simulink model "drawing_only"  (R2022b)
settings: Solver=VariableStepAuto  StartTime=0.0  StopTime=160  RelTol=1e-3
libraries: fl_lib x8, simulink x1
settings Model: Creator=Haposan  LastModifiedBy=Haposan

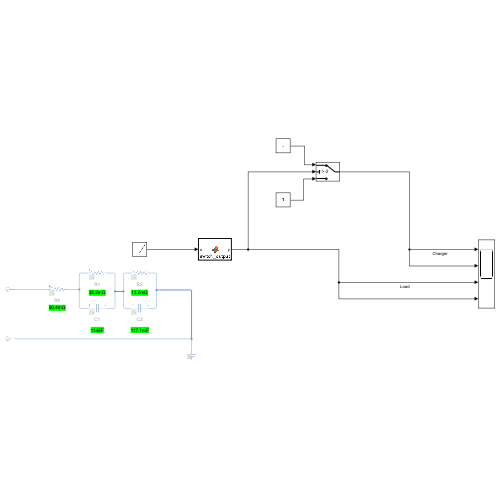
[thumbnail: Simulink's stored preview of the top-level diagram]
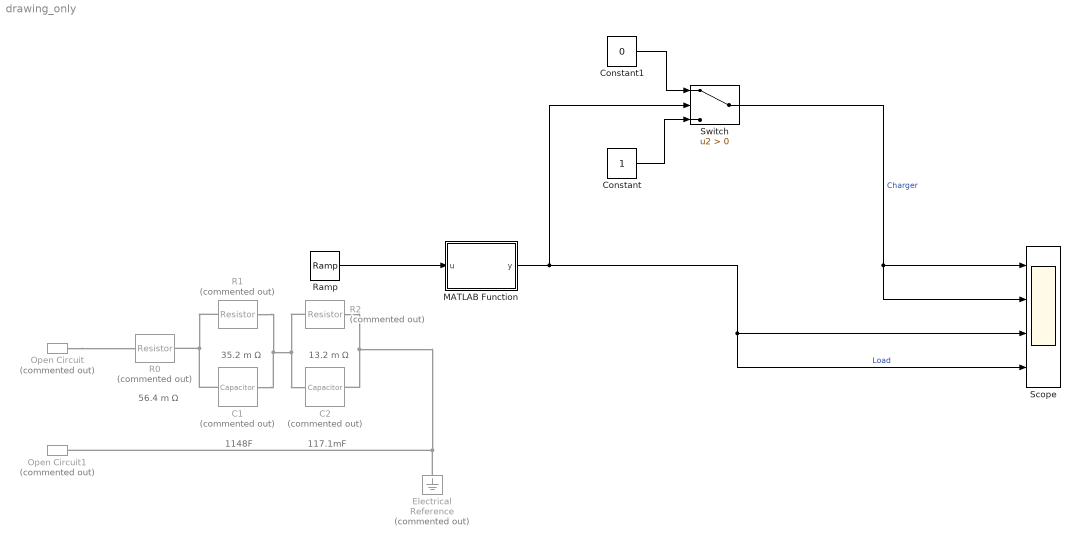
== system drawing_only ==
  note: 56.4 m Ω
  note: 13.2 m Ω
  note: 1148F
  note: 35.2 m Ω
  note: 117.1mF
  C1 : fl_lib/Electrical/Electrical Elements/Capacitor  Commented=on  c=1148 F  r=1e-6 Ohm  g=0 1/Ohm  i_specify=off  i_priority=None  i=0 A  i_nominal_specify=off  i_nominal_unit=A  i_nominal_value=1  v_specify=off  v_priority=None  v=0 V  v_nominal_specify=off  v_nominal_unit=V  v_nominal_value=1  vc_specify=off  vc_priority=High  vc=0 V  vc_nominal_specify=off  vc_nominal_unit=V  vc_nominal_value=1
  C2 : fl_lib/Electrical/Electrical Elements/Capacitor  Commented=on  c=117.1E-3 F  r=1e-6 Ohm  g=0 1/Ohm  i_specify=off  i_priority=None  i=0 A  i_nominal_specify=off  i_nominal_unit=A  i_nominal_value=1  v_specify=off  v_priority=None  v=0 V  v_nominal_specify=off  v_nominal_unit=V  v_nominal_value=1  vc_specify=off  vc_priority=High  vc=0 V  vc_nominal_specify=off  vc_nominal_unit=V  vc_nominal_value=1
  Constant : Constant
  Constant1 : Constant  Value=0
  Electrical Reference : fl_lib/Electrical/Electrical Elements/Electrical Reference  Commented=on
  MATLAB Function : MATLAB Function  TreatAsAtomicUnit=on
  Open Circuit : fl_lib/Electrical/Electrical Elements/Open Circuit  Commented=on  v_specify=off  v_priority=None  v=0 V  v_nominal_specify=off  v_nominal_unit=V  v_nominal_value=1
  Open Circuit1 : fl_lib/Electrical/Electrical Elements/Open Circuit  Commented=on  v_specify=off  v_priority=None  v=0 V  v_nominal_specify=off  v_nominal_unit=V  v_nominal_value=1
  R0 : fl_lib/Electrical/Electrical Elements/Resistor  Commented=on  R=56.4E-3 Ohm  i_specify=off  i_priority=None  i=0 A  i_nominal_specify=off  i_nominal_unit=A  i_nominal_value=1  v_specify=off  v_priority=None  v=0 V  v_nominal_specify=off  v_nominal_unit=V  v_nominal_value=1
  R1 : fl_lib/Electrical/Electrical Elements/Resistor  Commented=on  R=35.2E-3 Ohm  i_specify=off  i_priority=None  i=0 A  i_nominal_specify=off  i_nominal_unit=A  i_nominal_value=1  v_specify=off  v_priority=None  v=0 V  v_nominal_specify=off  v_nominal_unit=V  v_nominal_value=1
  R2 : fl_lib/Electrical/Electrical Elements/Resistor  Commented=on  R=13.2E-3 Ohm  i_specify=off  i_priority=None  i=0 A  i_nominal_specify=off  i_nominal_unit=A  i_nominal_value=1  v_specify=off  v_priority=None  v=0 V  v_nominal_specify=off  v_nominal_unit=V  v_nominal_value=1
  Ramp : simulink/Sources/Ramp  slope=1  start=0  InitialOutput=0
  Scope : Scope  NumInputPorts=4
  Switch : Switch  Criteria=u2 > Threshold  SaturateOnIntegerOverflow=off  InputSameDT=off
  wires:
  Switch/1 -> Scope/2, Scope/1  "Charger"
  Constant/1 -> Switch/3
  Constant1/1 -> Switch/1
  MATLAB Function/1(y) -> Switch/2, Scope/4, Scope/3  "Load"
  Ramp/1 -> MATLAB Function/1(u)
  connections:
  R1/RConn1 -- C1/RConn1 -- R2/LConn1 -- C2/LConn1
  C1/LConn1 -- R1/LConn1 -- R0/RConn1
  R2/RConn1 -- C2/RConn1 -- Electrical Reference/LConn1 -- Open Circuit1/LConn1
  Open Circuit/LConn1 -- R0/LConn1

== matlab function drawing_only/MATLAB Function ==
  data: u input; y output
function y = switch_output(u)
y = 0
    if u >= 99.5
        y = 1;
    elseif u <= 0.05
        y = 0;
    else
        y = y;  % keep the previous value of y
    end
end
